simulink library "Arithmetic_Operations_Lib"  (R2023a)
settings: Solver=ode45  StartTime=0.0  StopTime=10.0  RelTol=1e-3  EnableMultiTasking=on
libraries: Miscellaneous x202
(part 2 of 4)

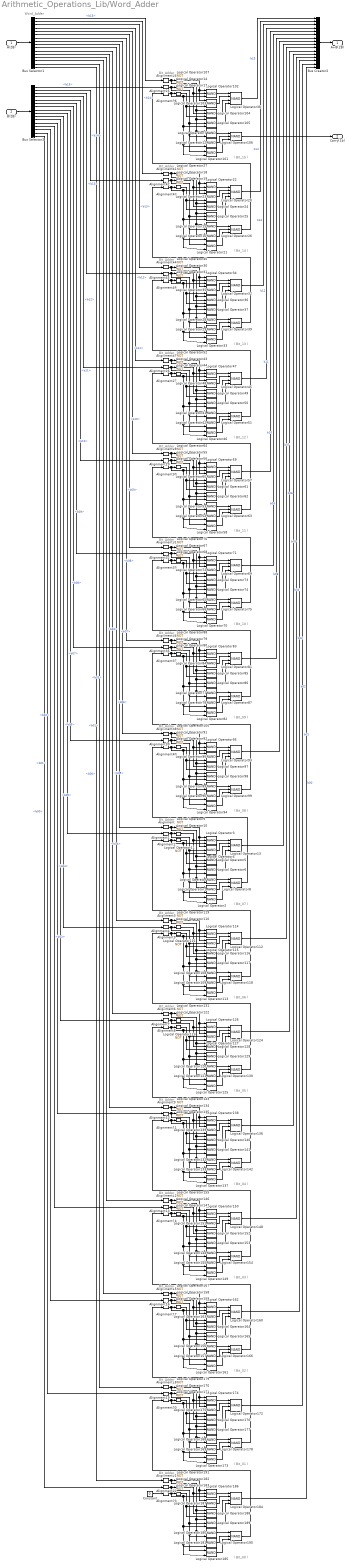
== system Arithmetic_Operations_Lib/Word_Adder ==
  note: Word_Adder
  note: Bit_Adder
  note: ( Bit_07 )
  note: Bit_Adder
  note: ( Bit_06 )
  note: Bit_Adder
  note: ( Bit_05 )
  note: Bit_Adder
  note: ( Bit_04 )
  note: Bit_Adder
  note: ( Bit_03 )
  note: Bit_Adder
  note: ( Bit_02 )
  note: Bit_Adder
  note: ( Bit_01 )
  note: Bit_Adder
  note: ( Bit_00 )
  note: ( Bit_13 )
  note: Bit_Adder
  note: Bit_Adder
  note: ( Bit_12 )
  note: ( Bit_11 )
  note: Bit_Adder
  note: ( Bit_10 )
  note: ( Bit_09 )
  note: Bit_Adder
  note: Bit_Adder
  note: ( Bit_08 )
  note: Bit_Adder
  note: ( Bit_14 )
  note: ( Bit_15 )
  note: Bit_Adder
  note: Bit_Adder
  A(2B) : Inport
  B(2B) : Inport  Port=2
  Alignment{,1..47} (48 alike) : Miscellaneous/Alignment  SystemSampleTime=-1  VariantActivationTime=update diagram  Latency=0  AutoFrameSizeCalculation=off
  Bus Creator2 : BusCreator  Inputs=16
  Bus Selector1 : BusSelector  OutputSignals=b15,b14,b13,b12,b11,b10,b09,b08,b07,b06,b05,b04,b03,b02,b01,b00
  Bus Selector2 : BusSelector  OutputSignals=b15,b14,b13,b12,b11,b10,b09,b08,b07,b06,b05,b04,b03,b02,b01,b00
  Constant : Constant  Value=0
  Logical Operator{,1..2,7,12,15..16,21,28..29,33,41..42,46,53..54,58,65..66,70,77..78,82,89..90,94,101,108..109,113,120..121,125,132..133,137,144..145,149,156..157,161,168..169,173,180..181,185} (48 alike) : Logic  Operator=NAND  IconShape=distinctive  AllPortsSameDT=off  OutDataTypeStr=boolean
  Logical Operator{9..11,14,17..19,27,30..31,40,43..44,52,55..56,64,67..68,76,79..80,88,91..92,100,107,110..111,119,122..123,131,134..135,143,146..147,155,158..159,167,170..171,179,182..183,191} (48 alike) : Logic  Operator=NOT  Inputs=4  IconShape=distinctive  AllPortsSameDT=off  OutDataTypeStr=boolean
  Logical Operator{3..6,8,22..26,34..37,39,47..51,59..63,71..75,83..87,95..99,102..106,114..118,126..130,138..142,150..154,162..166,174..178,186..190} (80 alike) : Logic  Operator=NAND  Inputs=3  IconShape=distinctive  AllPortsSameDT=off  OutDataTypeStr=boolean
  Logical Operator{13,20,32,38,45,57,69,81,93,112,124,136,148,160,172,184} (16 alike) : Logic  Operator=NAND  Inputs=4  IconShape=distinctive  AllPortsSameDT=off  OutDataTypeStr=boolean
  A+B(2B) : Outport
  Carry(1b) : Outport  Port=2
  wires:
  Bus Selector1/11 -> Alignment6/1  "<b05>"
  Bus Selector2/14 -> Alignment16/1  "<b02>"
  Bus Selector2/16 -> Alignment22/1  "<b00>"
  Bus Selector2/13 -> Alignment13/1  "<b03>"
  Bus Selector1/16 -> Alignment21/1  "<b00>"
  Bus Selector1/12 -> Alignment9/1  "<b04>"
  Bus Selector2/9 -> Alignment1/1  "<b07>"
  Bus Selector2/11 -> Alignment7/1  "<b05>"
  Bus Selector1/15 -> Alignment18/1  "<b01>"
  Bus Selector2/10 -> Alignment4/1  "<b06>"
  Logical Operator172/1 -> Bus Creator2/15  "b01"
  Logical Operator13/1 -> Bus Creator2/9  "b07"
  Bus Selector1/14 -> Alignment15/1  "<b02>"
  Logical Operator184/1 -> Bus Creator2/16  "b00"
  Logical Operator124/1 -> Bus Creator2/11  "b05"
  Bus Selector2/15 -> Alignment19/1  "<b01>"
  Logical Operator112/1 -> Bus Creator2/10  "b06"
  Logical Operator148/1 -> Bus Creator2/13  "b03"
  Bus Selector1/10 -> Alignment3/1  "<b06>"
  Logical Operator136/1 -> Bus Creator2/12  "b04"
  Bus Selector1/13 -> Alignment12/1  "<b03>"
  Logical Operator8/1 -> Alignment40/1
  Logical Operator160/1 -> Bus Creator2/14  "b02"
  Bus Selector1/9 -> Alignment/1  "<b07>"
  Bus Selector2/12 -> Alignment10/1  "<b04>"
  Logical Operator11/1 -> Logical Operator4/3, Logical Operator5/3
  Logical Operator10/1 -> Logical Operator3/2, Logical Operator5/2
  Logical Operator9/1 -> Logical Operator4/1, Logical Operator3/1
  Logical Operator118/1 -> Alignment2/1
  Logical Operator2/1 -> Logical Operator8/3
  Logical Operator1/1 -> Logical Operator8/2
  Logical Operator/1 -> Logical Operator8/1
  Logical Operator6/1 -> Logical Operator13/4
  Logical Operator5/1 -> Logical Operator13/3
  Logical Operator4/1 -> Logical Operator13/2
  Logical Operator3/1 -> Logical Operator13/1
  Alignment/1 -> Logical Operator9/1, Logical Operator5/1, Logical Operator6/1, Logical Operator/1, Logical Operator1/1
  Alignment1/1 -> Logical Operator4/2, Logical Operator6/2, Logical Operator/2, Logical Operator2/1, Logical Operator10/1
  Alignment2/1 -> Logical Operator3/3, Logical Operator6/3, Logical Operator1/2, Logical Operator2/2, Logical Operator11/1
  Logical Operator111/1 -> Logical Operator115/3, Logical Operator116/3
  Logical Operator110/1 -> Logical Operator114/2, Logical Operator116/2
  Logical Operator119/1 -> Logical Operator115/1, Logical Operator114/1
  Logical Operator130/1 -> Alignment5/1
  Logical Operator113/1 -> Logical Operator118/3
  Logical Operator109/1 -> Logical Operator118/2
  Logical Operator108/1 -> Logical Operator118/1
  Logical Operator117/1 -> Logical Operator112/4
  Logical Operator116/1 -> Logical Operator112/3
  Logical Operator115/1 -> Logical Operator112/2
  Logical Operator114/1 -> Logical Operator112/1
  Alignment3/1 -> Logical Operator119/1, Logical Operator109/1, Logical Operator108/1, Logical Operator117/1, Logical Operator116/1
  Alignment4/1 -> Logical Operator115/2, Logical Operator117/2, Logical Operator108/2, Logical Operator113/1, Logical Operator110/1
  Alignment5/1 -> Logical Operator114/3, Logical Operator117/3, Logical Operator109/2, Logical Operator113/2, Logical Operator111/1
  Logical Operator123/1 -> Logical Operator127/3, Logical Operator128/3
  Logical Operator122/1 -> Logical Operator126/2, Logical Operator128/2
  Logical Operator131/1 -> Logical Operator127/1, Logical Operator126/1
  Logical Operator142/1 -> Alignment8/1
  Logical Operator125/1 -> Logical Operator130/3
  Logical Operator121/1 -> Logical Operator130/2
  Logical Operator120/1 -> Logical Operator130/1
  Logical Operator129/1 -> Logical Operator124/4
  Logical Operator128/1 -> Logical Operator124/3
  Logical Operator127/1 -> Logical Operator124/2
  Logical Operator126/1 -> Logical Operator124/1
  Alignment6/1 -> Logical Operator131/1, Logical Operator121/1, Logical Operator120/1, Logical Operator129/1, Logical Operator128/1
  Alignment7/1 -> Logical Operator125/1, Logical Operator120/2, Logical Operator129/2, Logical Operator127/2, Logical Operator122/1
  Alignment8/1 -> Logical Operator126/3, Logical Operator129/3, Logical Operator121/2, Logical Operator125/2, Logical Operator123/1
  Logical Operator135/1 -> Logical Operator139/3, Logical Operator140/3
  Logical Operator134/1 -> Logical Operator138/2, Logical Operator140/2
  Logical Operator143/1 -> Logical Operator139/1, Logical Operator138/1
  Logical Operator154/1 -> Alignment11/1
  Logical Operator137/1 -> Logical Operator142/3
  Logical Operator133/1 -> Logical Operator142/2
  Logical Operator132/1 -> Logical Operator142/1
  Logical Operator141/1 -> Logical Operator136/4
  Logical Operator140/1 -> Logical Operator136/3
  Logical Operator139/1 -> Logical Operator136/2
  Logical Operator138/1 -> Logical Operator136/1
  Alignment9/1 -> Logical Operator143/1, Logical Operator140/1, Logical Operator141/1, Logical Operator132/1, Logical Operator133/1
  Alignment10/1 -> Logical Operator139/2, Logical Operator141/2, Logical Operator132/2, Logical Operator137/1, Logical Operator134/1
  Alignment11/1 -> Logical Operator138/3, Logical Operator141/3, Logical Operator133/2, Logical Operator137/2, Logical Operator135/1
  Logical Operator147/1 -> Logical Operator151/3, Logical Operator152/3
  Logical Operator146/1 -> Logical Operator150/2, Logical Operator152/2
  Logical Operator155/1 -> Logical Operator151/1, Logical Operator150/1
  Logical Operator166/1 -> Alignment14/1
  Logical Operator149/1 -> Logical Operator154/3
  Logical Operator145/1 -> Logical Operator154/2
  Logical Operator144/1 -> Logical Operator154/1
  Logical Operator153/1 -> Logical Operator148/4
  Logical Operator152/1 -> Logical Operator148/3
  Logical Operator151/1 -> Logical Operator148/2
  Logical Operator150/1 -> Logical Operator148/1
  Alignment12/1 -> Logical Operator155/1, Logical Operator152/1, Logical Operator153/1, Logical Operator144/1, Logical Operator145/1
  Alignment13/1 -> Logical Operator151/2, Logical Operator153/2, Logical Operator144/2, Logical Operator149/1, Logical Operator146/1
  Alignment14/1 -> Logical Operator150/3, Logical Operator153/3, Logical Operator145/2, Logical Operator149/2, Logical Operator147/1
  Logical Operator159/1 -> Logical Operator163/3, Logical Operator164/3
  Logical Operator158/1 -> Logical Operator162/2, Logical Operator164/2
  Logical Operator167/1 -> Logical Operator163/1, Logical Operator162/1
  Logical Operator178/1 -> Alignment17/1
  Logical Operator161/1 -> Logical Operator166/3
  Logical Operator157/1 -> Logical Operator166/2
  Logical Operator156/1 -> Logical Operator166/1
  Logical Operator165/1 -> Logical Operator160/4
  Logical Operator164/1 -> Logical Operator160/3
  Logical Operator163/1 -> Logical Operator160/2
  Logical Operator162/1 -> Logical Operator160/1
  Alignment15/1 -> Logical Operator167/1, Logical Operator164/1, Logical Operator165/1, Logical Operator156/1, Logical Operator157/1
  Alignment16/1 -> Logical Operator163/2, Logical Operator165/2, Logical Operator156/2, Logical Operator161/1, Logical Operator158/1
  Alignment17/1 -> Logical Operator162/3, Logical Operator165/3, Logical Operator157/2, Logical Operator161/2, Logical Operator159/1
  Logical Operator171/1 -> Logical Operator175/3, Logical Operator176/3
  Logical Operator170/1 -> Logical Operator174/2, Logical Operator176/2
  Logical Operator179/1 -> Logical Operator175/1, Logical Operator174/1
  Logical Operator190/1 -> Alignment20/1
  Logical Operator173/1 -> Logical Operator178/3
  Logical Operator169/1 -> Logical Operator178/2
  Logical Operator168/1 -> Logical Operator178/1
  Logical Operator177/1 -> Logical Operator172/4
  Logical Operator176/1 -> Logical Operator172/3
  Logical Operator175/1 -> Logical Operator172/2
  Logical Operator174/1 -> Logical Operator172/1
  Alignment18/1 -> Logical Operator179/1, Logical Operator176/1, Logical Operator177/1, Logical Operator168/1, Logical Operator169/1
  Alignment19/1 -> Logical Operator175/2, Logical Operator177/2, Logical Operator168/2, Logical Operator173/1, Logical Operator170/1
  Alignment20/1 -> Logical Operator174/3, Logical Operator177/3, Logical Operator169/2, Logical Operator173/2, Logical Operator171/1
  Logical Operator183/1 -> Logical Operator187/3, Logical Operator188/3
  Logical Operator182/1 -> Logical Operator186/2, Logical Operator188/2
  Logical Operator191/1 -> Logical Operator187/1, Logical Operator186/1
  Constant/1 -> Alignment23/1
  Logical Operator185/1 -> Logical Operator190/3
  Logical Operator181/1 -> Logical Operator190/2
  Logical Operator180/1 -> Logical Operator190/1
  Logical Operator189/1 -> Logical Operator184/4
  Logical Operator188/1 -> Logical Operator184/3
  Logical Operator187/1 -> Logical Operator184/2
  Logical Operator186/1 -> Logical Operator184/1
  Alignment21/1 -> Logical Operator191/1, Logical Operator188/1, Logical Operator189/1, Logical Operator180/1, Logical Operator181/1
  Alignment22/1 -> Logical Operator187/2, Logical Operator189/2, Logical Operator180/2, Logical Operator185/1, Logical Operator182/1
  Alignment23/1 -> Logical Operator186/3, Logical Operator189/3, Logical Operator181/2, Logical Operator185/2, Logical Operator183/1
  Bus Creator2/1 -> A+B(2B)/1
  Logical Operator79/1 -> Logical Operator83/2, Logical Operator85/2
  Alignment28/1 -> Logical Operator64/1, Logical Operator61/1, Logical Operator62/1, Logical Operator53/1, Logical Operator54/1
  Logical Operator56/1 -> Logical Operator60/3, Logical Operator61/3
  Logical Operator65/1 -> Logical Operator75/1
  Alignment43/1 -> Logical Operator22/3, Logical Operator25/3, Logical Operator16/2, Logical Operator21/2, Logical Operator19/1
  Logical Operator90/1 -> Logical Operator99/2
  Logical Operator100/1 -> Logical Operator96/1, Logical Operator95/1
  Alignment33/1 -> Logical Operator71/3, Logical Operator74/3, Logical Operator66/2, Logical Operator70/2, Logical Operator68/1
  Logical Operator33/1 -> Logical Operator39/3
  Logical Operator24/1 -> Logical Operator20/3
  Alignment35/1 -> Logical Operator84/2, Logical Operator86/2, Logical Operator77/2, Logical Operator82/1, Logical Operator79/1
  Logical Operator85/1 -> Logical Operator81/3
  Logical Operator58/1 -> Logical Operator63/3
  Logical Operator82/1 -> Logical Operator87/3
  Logical Operator36/1 -> Logical Operator32/3
  Logical Operator83/1 -> Logical Operator81/1
  Alignment24/1 -> Logical Operator107/1, Logical Operator104/1, Logical Operator105/1, Logical Operator7/1, Logical Operator12/1
  Logical Operator80/1 -> Logical Operator84/3, Logical Operator85/3
  Logical Operator47/1 -> Logical Operator45/1
  Logical Operator104/1 -> Logical Operator38/3
  Logical Operator60/1 -> Logical Operator57/2
  Logical Operator74/1 -> Logical Operator69/4
  Alignment30/1 -> Logical Operator59/3, Logical Operator62/3, Logical Operator54/2, Logical Operator58/2, Logical Operator56/1
  Logical Operator64/1 -> Logical Operator60/1, Logical Operator59/1
  Logical Operator51/1 -> Alignment46/1
  Logical Operator71/1 -> Logical Operator69/1
  Logical Operator87/1 -> Alignment33/1
  Logical Operator39/1 -> Alignment43/1
  Logical Operator66/1 -> Logical Operator75/2
  Logical Operator70/1 -> Logical Operator75/3
  Alignment47/1 -> Logical Operator52/1, Logical Operator49/1, Logical Operator50/1, Logical Operator41/1, Logical Operator42/1
  Alignment45/1 -> Logical Operator33/1, Logical Operator28/2, Logical Operator37/2, Logical Operator35/2, Logical Operator30/1
  Logical Operator67/1 -> Logical Operator71/2, Logical Operator73/2
  Logical Operator18/1 -> Logical Operator22/2, Logical Operator24/2
  Alignment29/1 -> Logical Operator60/2, Logical Operator62/2, Logical Operator53/2, Logical Operator58/1, Logical Operator55/1
  Logical Operator103/1 -> Logical Operator38/2
  Alignment27/1 -> Logical Operator47/3, Logical Operator50/3, Logical Operator42/2, Logical Operator46/2, Logical Operator44/1
  Logical Operator76/1 -> Logical Operator72/1, Logical Operator71/1
  Logical Operator41/1 -> Logical Operator51/1
  Alignment46/1 -> Logical Operator34/3, Logical Operator37/3, Logical Operator29/2, Logical Operator33/2, Logical Operator31/1
  Logical Operator14/1 -> Logical Operator102/2, Logical Operator104/2
  Logical Operator62/1 -> Logical Operator57/4
  Logical Operator105/1 -> Logical Operator38/4
  Logical Operator75/1 -> Alignment30/1
  Logical Operator28/1 -> Logical Operator39/1
  Logical Operator55/1 -> Logical Operator59/2, Logical Operator61/2
  Logical Operator26/1 -> Alignment36/1
  Alignment41/1 -> Logical Operator27/1, Logical Operator16/1, Logical Operator15/1, Logical Operator25/1, Logical Operator24/1
  Logical Operator50/1 -> Logical Operator45/4
  Logical Operator43/1 -> Logical Operator47/2, Logical Operator49/2
  Logical Operator44/1 -> Logical Operator48/3, Logical Operator49/3
  Logical Operator46/1 -> Logical Operator51/3
  Logical Operator52/1 -> Logical Operator48/1, Logical Operator47/1
  Logical Operator48/1 -> Logical Operator45/2
  Logical Operator49/1 -> Logical Operator45/3
  Logical Operator63/1 -> Alignment27/1
  Alignment44/1 -> Logical Operator40/1, Logical Operator29/1, Logical Operator28/1, Logical Operator37/1, Logical Operator36/1
  Logical Operator12/1 -> Logical Operator106/2
  Logical Operator29/1 -> Logical Operator39/2
  Logical Operator40/1 -> Logical Operator35/1, Logical Operator34/1
  Logical Operator35/1 -> Logical Operator32/2
  Logical Operator53/1 -> Logical Operator63/1
  Logical Operator37/1 -> Logical Operator32/4
  Logical Operator72/1 -> Logical Operator69/2
  Logical Operator59/1 -> Logical Operator57/1
  Logical Operator107/1 -> Logical Operator103/1, Logical Operator102/1
  Logical Operator99/1 -> Alignment37/1
  Logical Operator102/1 -> Logical Operator38/1
  Logical Operator31/1 -> Logical Operator35/3, Logical Operator36/3
  Logical Operator95/1 -> Logical Operator93/1
  Logical Operator22/1 -> Logical Operator20/1
  Alignment42/1 -> Logical Operator23/2, Logical Operator25/2, Logical Operator15/2, Logical Operator21/1, Logical Operator18/1
  Alignment31/1 -> Logical Operator76/1, Logical Operator73/1, Logical Operator74/1, Logical Operator65/1, Logical Operator66/1
  Logical Operator23/1 -> Logical Operator20/2
  Logical Operator89/1 -> Logical Operator99/1
  Logical Operator42/1 -> Logical Operator51/2
  Alignment36/1 -> Logical Operator102/3, Logical Operator105/3, Logical Operator12/2, Logical Operator101/2, Logical Operator17/1
  Logical Operator25/1 -> Logical Operator20/4
  Logical Operator15/1 -> Logical Operator26/1
  Logical Operator7/1 -> Logical Operator106/1
  Logical Operator27/1 -> Logical Operator23/1, Logical Operator22/1
  Logical Operator19/1 -> Logical Operator23/3, Logical Operator24/3
  Alignment25/1 -> Logical Operator103/2, Logical Operator105/2, Logical Operator7/2, Logical Operator101/1, Logical Operator14/1
  Logical Operator17/1 -> Logical Operator103/3, Logical Operator104/3
  Logical Operator30/1 -> Logical Operator34/2, Logical Operator36/2
  Logical Operator34/1 -> Logical Operator32/1
  Logical Operator78/1 -> Logical Operator87/2
  Logical Operator98/1 -> Logical Operator93/4
  Alignment37/1 -> Logical Operator83/3, Logical Operator86/3, Logical Operator78/2, Logical Operator82/2, Logical Operator80/1
  Alignment26/1 -> Logical Operator48/2, Logical Operator50/2, Logical Operator41/2, Logical Operator46/1, Logical Operator43/1
  Logical Operator94/1 -> Logical Operator99/3
  Logical Operator21/1 -> Logical Operator26/3
  Alignment34/1 -> Logical Operator88/1, Logical Operator85/1, Logical Operator86/1, Logical Operator77/1, Logical Operator78/1
  Logical Operator61/1 -> Logical Operator57/3
  Logical Operator96/1 -> Logical Operator93/2
  Logical Operator97/1 -> Logical Operator93/3
  Alignment38/1 -> Logical Operator100/1, Logical Operator97/1, Logical Operator98/1, Logical Operator89/1, Logical Operator90/1
  Alignment32/1 -> Logical Operator72/2, Logical Operator74/2, Logical Operator65/2, Logical Operator70/1, Logical Operator67/1
  Logical Operator91/1 -> Logical Operator95/2, Logical Operator97/2
  Logical Operator88/1 -> Logical Operator84/1, Logical Operator83/1
  Logical Operator68/1 -> Logical Operator72/3, Logical Operator73/3
  Logical Operator73/1 -> Logical Operator69/3
  Logical Operator101/1 -> Logical Operator106/3
  Alignment40/1 -> Logical Operator95/3, Logical Operator98/3, Logical Operator90/2, Logical Operator94/2, Logical Operator92/1
  Logical Operator92/1 -> Logical Operator96/3, Logical Operator97/3
  Logical Operator16/1 -> Logical Operator26/2
  Logical Operator54/1 -> Logical Operator63/2
  Alignment39/1 -> Logical Operator96/2, Logical Operator98/2, Logical Operator89/2, Logical Operator94/1, Logical Operator91/1
  Logical Operator84/1 -> Logical Operator81/2
  Logical Operator77/1 -> Logical Operator87/1
  Logical Operator86/1 -> Logical Operator81/4
  Logical Operator38/1 -> Bus Creator2/1  "b15"
  Logical Operator20/1 -> Bus Creator2/2  "b14"
  Logical Operator32/1 -> Bus Creator2/3  "b13"
  Logical Operator45/1 -> Bus Creator2/4  "b12"
  Logical Operator57/1 -> Bus Creator2/5  "b11"
  Logical Operator69/1 -> Bus Creator2/6  "b10"
  Logical Operator81/1 -> Bus Creator2/7  "b09"
  Logical Operator93/1 -> Bus Creator2/8  "b08"
  Bus Selector2/8 -> Alignment39/1  "<b08>"
  Bus Selector2/7 -> Alignment35/1  "<b09>"
  Bus Selector2/6 -> Alignment32/1  "<b10>"
  Bus Selector2/5 -> Alignment29/1  "<b11>"
  Bus Selector2/4 -> Alignment26/1  "<b12>"
  Bus Selector2/3 -> Alignment45/1  "<b13>"
  Bus Selector2/2 -> Alignment42/1  "<b14>"
  Bus Selector2/1 -> Alignment25/1  "<b15>"
  Bus Selector1/8 -> Alignment38/1  "<b08>"
  Bus Selector1/7 -> Alignment34/1  "<b09>"
  Bus Selector1/6 -> Alignment31/1  "<b10>"
  Bus Selector1/5 -> Alignment28/1  "<b11>"
  Bus Selector1/4 -> Alignment47/1  "<b12>"
  Bus Selector1/3 -> Alignment44/1  "<b13>"
  Bus Selector1/2 -> Alignment41/1  "<b14>"
  Bus Selector1/1 -> Alignment24/1  "<b15>"
  A(2B)/1 -> Bus Selector1/1
  B(2B)/1 -> Bus Selector2/1
  Logical Operator106/1 -> Carry(1b)/1
